simulink library "controller_Lib"  (R2020a)
settings: Solver=VariableStepAuto  StartTime=0.0  StopTime=10.0  RelTol=1e-3
settings Model: Creator=NIKITA  LastModifiedBy=NIKITA

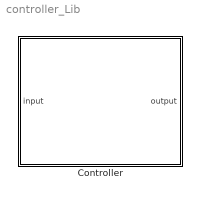
== system controller_Lib ==
  Controller : Subsystem  mask{Kp=36, Ki=4, Ts=0.01}
      mask Display: image('IC.jpg'); % Use "Edit Image" on toolstrip to change.

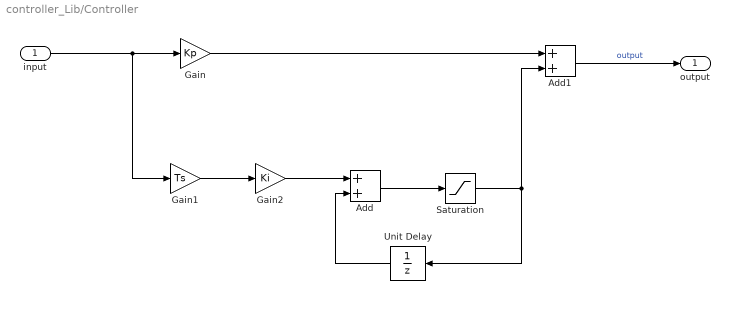
== system controller_Lib/Controller ==
  input : Inport
  Add : Sum
  Add1 : Sum
  Gain : Gain  Gain=Kp
  Gain1 : Gain  Gain=Ts
  Gain2 : Gain  Gain=Ki
  Saturation : Saturate  UpperLimit=1  LowerLimit=-1
  Unit Delay : UnitDelay  SampleTime=-1  HasFrameUpgradeWarning=on
  output : Outport
  wires:
  Unit Delay/1 -> Add/2
  Saturation/1 -> Unit Delay/1, Add1/2
  Gain2/1 -> Add/1
  input/1 -> Gain1/1, Gain/1
  Gain/1 -> Add1/1
  Gain1/1 -> Gain2/1
  Add/1 -> Saturation/1
  Add1/1 -> output/1  "output"
